simulink model "Aplicatia_1"  (R2017b)
settings: Solver=ode4  StartTime=0.0  StopTime=4  FixedStep=0.01  RelTol=1e-3
libraries: simulink x6
settings Model: Creator=tutuc  LastModifiedBy=tutuc

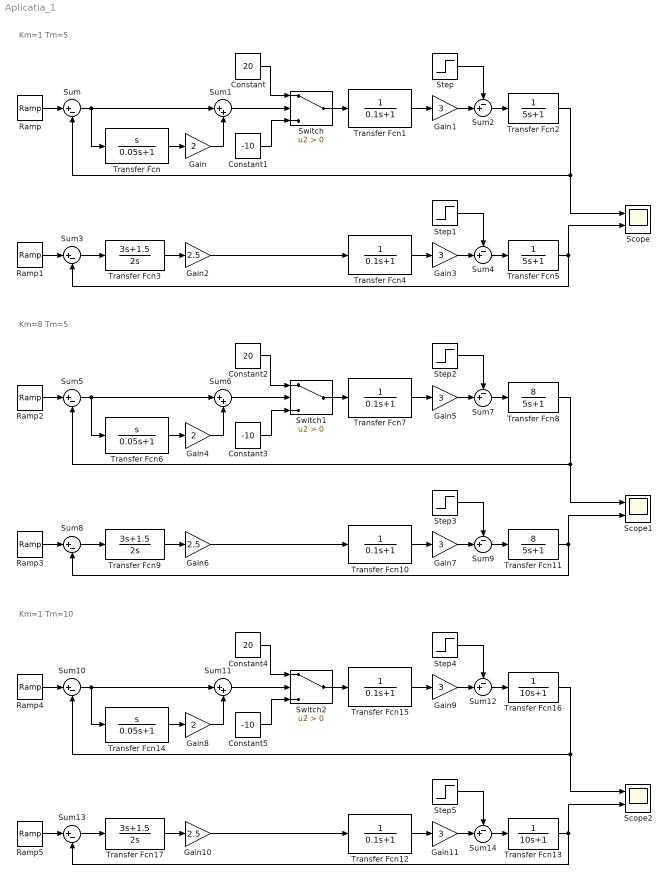
== system Aplicatia_1 ==
  note: Km=1 Tm=5
  note: Km=8 Tm=5
  note: Km=1 Tm=10
  Constant : Constant  Value=20
  Constant1 : Constant  Value=-10
  Constant2 : Constant  Value=20
  Constant3 : Constant  Value=-10
  Constant4 : Constant  Value=20
  Constant5 : Constant  Value=-10
  Gain : Gain  Gain=2
  Gain{1,3,5,7,9,11} (6 alike) : Gain  Gain=3
  Gain10 : Gain  Gain=2.5
  Gain2 : Gain  Gain=2.5
  Gain4 : Gain  Gain=2
  Gain6 : Gain  Gain=2.5
  Gain8 : Gain  Gain=2
  Ramp{,1..5} (6 alike) : simulink/Sources/Ramp  slope=2  start=0  X0=0
  Scope : Scope  NumInputPorts=2
  Scope1 : Scope  NumInputPorts=2
  Scope2 : Scope  NumInputPorts=2
  Step{,1..5} (6 alike) : Step  Time=2.5  After=15  SampleTime=0
  Sum{,3,5,8,10,13} (6 alike) : Sum  Inputs=|+-
  Sum1 : Sum  Inputs=|++
  Sum11 : Sum  Inputs=|++
  Sum{2,4,7,9,12,14} (6 alike) : Sum  Inputs=-+|
  Sum6 : Sum  Inputs=|++
  Switch : Switch  Criteria=u2 > Threshold
  Switch1 : Switch  Criteria=u2 > Threshold
  Switch2 : Switch  Criteria=u2 > Threshold
  Transfer Fcn : TransferFcn  Numerator=[1 0]  Denominator=[0.05 1]
  Transfer Fcn{1,4,7,10,12,15} (6 alike) : TransferFcn  Denominator=[0.1 1]
  Transfer Fcn11 : TransferFcn  Numerator=[8]  Denominator=[5 1]
  Transfer Fcn13 : TransferFcn  Denominator=[10 1]
  Transfer Fcn14 : TransferFcn  Numerator=[1 0]  Denominator=[0.05 1]
  Transfer Fcn16 : TransferFcn  Denominator=[10 1]
  Transfer Fcn17 : TransferFcn  Numerator=[3 1.5]  Denominator=[2 0]
  Transfer Fcn2 : TransferFcn  Denominator=[5 1]
  Transfer Fcn3 : TransferFcn  Numerator=[3 1.5]  Denominator=[2 0]
  Transfer Fcn5 : TransferFcn  Denominator=[5 1]
  Transfer Fcn6 : TransferFcn  Numerator=[1 0]  Denominator=[0.05 1]
  Transfer Fcn8 : TransferFcn  Numerator=[8]  Denominator=[5 1]
  Transfer Fcn9 : TransferFcn  Numerator=[3 1.5]  Denominator=[2 0]
  wires:
  Ramp/1 -> Sum/1
  Transfer Fcn/1 -> Gain/1
  Gain/1 -> Sum1/2
  Sum/1 -> Transfer Fcn/1, Sum1/1
  Sum1/1 -> Switch/2
  Constant/1 -> Switch/1
  Constant1/1 -> Switch/3
  Switch/1 -> Transfer Fcn1/1
  Transfer Fcn1/1 -> Gain1/1
  Gain1/1 -> Sum2/2
  Step/1 -> Sum2/1
  Sum2/1 -> Transfer Fcn2/1
  Transfer Fcn2/1 -> Scope/1, Sum/2
  Ramp1/1 -> Sum3/1
  Sum3/1 -> Transfer Fcn3/1
  Transfer Fcn3/1 -> Gain2/1
  Sum4/1 -> Transfer Fcn5/1
  Step1/1 -> Sum4/1
  Gain3/1 -> Sum4/2
  Transfer Fcn4/1 -> Gain3/1
  Gain2/1 -> Transfer Fcn4/1
  Transfer Fcn5/1 -> Scope/2, Sum3/2
  Transfer Fcn11/1 -> Sum8/2, Scope1/2
  Gain6/1 -> Transfer Fcn10/1
  Transfer Fcn10/1 -> Gain7/1
  Gain7/1 -> Sum9/2
  Step3/1 -> Sum9/1
  Sum9/1 -> Transfer Fcn11/1
  Transfer Fcn9/1 -> Gain6/1
  Sum8/1 -> Transfer Fcn9/1
  Ramp3/1 -> Sum8/1
  Transfer Fcn8/1 -> Sum5/2, Scope1/1
  Sum7/1 -> Transfer Fcn8/1
  Step2/1 -> Sum7/1
  Gain5/1 -> Sum7/2
  Transfer Fcn7/1 -> Gain5/1
  Switch1/1 -> Transfer Fcn7/1
  Constant3/1 -> Switch1/3
  Constant2/1 -> Switch1/1
  Sum6/1 -> Switch1/2
  Sum5/1 -> Sum6/1, Transfer Fcn6/1
  Gain4/1 -> Sum6/2
  Transfer Fcn6/1 -> Gain4/1
  Ramp2/1 -> Sum5/1
  Ramp4/1 -> Sum10/1
  Transfer Fcn14/1 -> Gain8/1
  Gain8/1 -> Sum11/2
  Sum10/1 -> Transfer Fcn14/1, Sum11/1
  Sum11/1 -> Switch2/2
  Constant4/1 -> Switch2/1
  Constant5/1 -> Switch2/3
  Switch2/1 -> Transfer Fcn15/1
  Transfer Fcn15/1 -> Gain9/1
  Gain9/1 -> Sum12/2
  Step4/1 -> Sum12/1
  Sum12/1 -> Transfer Fcn16/1
  Transfer Fcn16/1 -> Scope2/1, Sum10/2
  Ramp5/1 -> Sum13/1
  Sum13/1 -> Transfer Fcn17/1
  Transfer Fcn17/1 -> Gain10/1
  Sum14/1 -> Transfer Fcn13/1
  Step5/1 -> Sum14/1
  Gain11/1 -> Sum14/2
  Transfer Fcn12/1 -> Gain11/1
  Gain10/1 -> Transfer Fcn12/1
  Transfer Fcn13/1 -> Scope2/2, Sum13/2
